simulink model "SIMULINK_MODEL"  (R2021b)
settings: Solver=VariableStepAuto  StartTime=0.0  StopTime=10.0  RelTol=1e-3
settings Model: Creator=Maheswaran  LastModifiedBy=Maheswaran

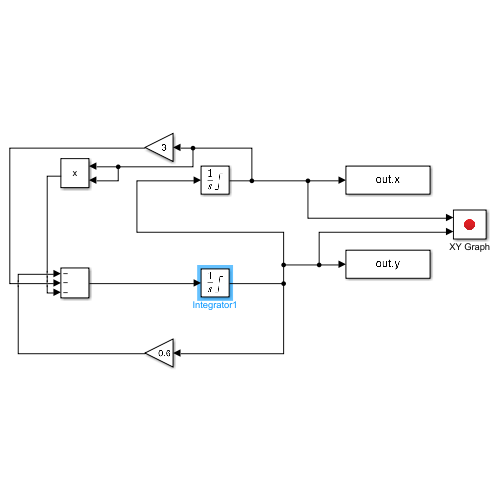
[thumbnail: Simulink's stored preview of the top-level diagram]
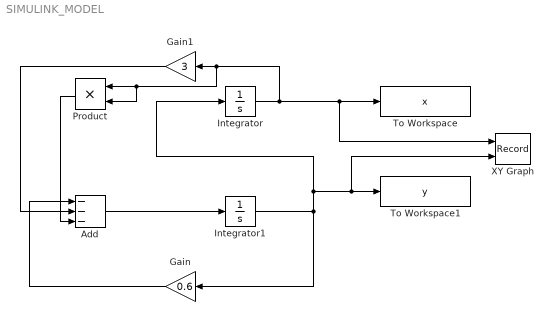
== system SIMULINK_MODEL ==
  Add : Sum  Inputs=---
  Gain : Gain  Gain=0.6
  Gain1 : Gain  Gain=3
  Integrator : Integrator  InitialCondition=-4  LimitOutput=on  UpperSaturationLimit=12  LowerSaturationLimit=-12
  Integrator1 : Integrator  InitialCondition=1  LimitOutput=on  UpperSaturationLimit=12  LowerSaturationLimit=-12
  Product : Product
  To Workspace : ToWorkspace  VariableName=x  SaveFormat=Timeseries  SampleTime=-1
  To Workspace1 : ToWorkspace  VariableName=y  SaveFormat=Timeseries  SampleTime=-1
  XY Graph : Record  FileSettingsInternal="{\"entries\":[{\"content\":{\"excelSettings\":{\"content\":{},\"type\":\"Streamout.ExcelSettings\"}},\"type\":\"Streamout.FileSettingStorage\",\"uuid\":\"46ca6a8e-a67a-4a63-81d4-74d655ba9dc1\"}],\"packageUris\":[\"http://schema.mathworks.com/mf0/streamout_blocks/R2020a\"],\"version\":\"1.0\"}"  Layout=[1 1]  SignalsInternal="{\"entries\":[{\"content\":{\"signals\":[{\"content\":{\"blockPath\":[\"SIMULINK_MODEL/XY Graph\"],\"channel\":[],\"dimensions\":[1],\"domain\":\"SIMULINK_MODEL/XY Graph\",\"lineColor\":\"#a2142f\",\"plots\":[1],\"port\":1,\"sid\":[\"\"],\"signalID\":192,\"signalName\":\"Integrator\"},\"type\":\"RecordBlkView.Signal\",\"uuid\":\"72aafa9a-5f44-4573-92f9-64460758b16e\"},{\"content\":{\"blockPath\":[\"SIMULINK_MODEL/XY Graph\"],\"channel\":[],\"dimensions\":[1],\"domain\":\"SIMULINK_MODEL/XY Graph\",\"lineColor\":\"#139fff\",\"plots\":[1],\"port\":2,\"sid\":[\"\"],\"signalID\":196,\"signalName\":\"Integrator1\"},\"type\":\"RecordBlkView.Signal\",\"uuid\":\"e09e1328-8571-41a5-903f-1a437328b668\"}]},\"type\":\"RecordBlkView.InputSignals\",\"uuid\":\"85dccb64-421e-4979-aab7-2c96188c6148\"}],\"packageUris\":[\"http://schema.mathworks.com/mf0/streamout_blocks/R2020a\"],\"version\":\"1.0\"}"  VisualizationBindings="{\"xyplotplugin\":{\"info\":[{\"series\":[{\"bindingParametersList\":[{\"parameter\":\"X-Axis\",\"signalID\":192,\"signalName\":\"Integrator\"},{\"parameter\":\"Y-Axis\",\"signalID\":196,\"signalName\":\"Integrator1\"}],\"seriesID\":29358}],\"subplotID\":1}]}}"  CompatibilityTag=XY
  wires:
  Integrator1/1 -> Integrator/1, XY Graph/2, To Workspace1/1, Gain/1
  Gain/1 -> Add/1
  Integrator/1 -> XY Graph/1, To Workspace/1, Gain1/1, Product/2, Product/1
  Gain1/1 -> Add/2
  Product/1 -> Add/3
  Add/1 -> Integrator1/1
